simulink model "ex1"  (R2020a)
settings: Solver=VariableStepAuto  StartTime=0.0  StopTime=10.0  RelTol=1e-3
undefined symbols (not defined in the file or in its folder): DiscIntNeverNeededParam, dz, nz
libraries: simulink x1

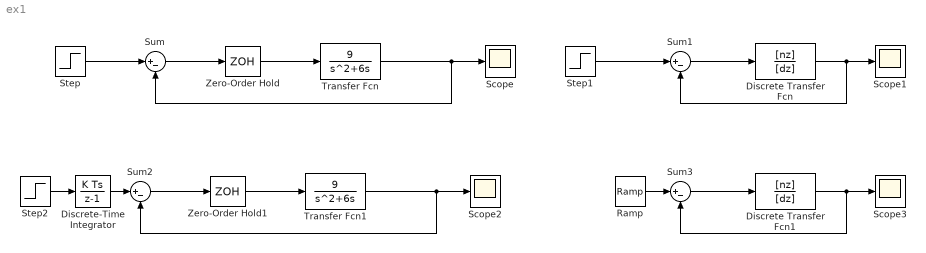
== system ex1 ==
  Discrete Transfer Fcn : DiscreteTransferFcn  Numerator=[nz]  Denominator=[dz]  SampleTime=0.1
  Discrete Transfer Fcn1 : DiscreteTransferFcn  Numerator=[nz]  Denominator=[dz]  SampleTime=0.1
  Discrete-Time Integrator : DiscreteIntegrator  SampleTime=-1  ICPrevOutput=DiscIntNeverNeededParam  ICPrevScaledInput=DiscIntNeverNeededParam
  Ramp : simulink/Sources/Ramp  slope=1  start=0  InitialOutput=0
  Scope{,1..3} (4 alike) : Scope
  Step : Step  SampleTime=0.1
  Step1 : Step  SampleTime=0.1
  Step2 : Step  SampleTime=0.1
  Sum{,1..3} (4 alike) : Sum  Inputs=|+-  SampleTime=0.1
  Transfer Fcn : TransferFcn  Numerator=[9]  Denominator=[1 6 0]
  Transfer Fcn1 : TransferFcn  Numerator=[9]  Denominator=[1 6 0]
  Zero-Order Hold : ZeroOrderHold  SampleTime=-1
  Zero-Order Hold1 : ZeroOrderHold  SampleTime=-1
  wires:
  Zero-Order Hold/1 -> Transfer Fcn/1
  Step/1 -> Sum/1
  Sum/1 -> Zero-Order Hold/1
  Transfer Fcn/1 -> Sum/2, Scope/1
  Step1/1 -> Sum1/1
  Sum1/1 -> Discrete Transfer Fcn/1
  Discrete Transfer Fcn/1 -> Sum1/2, Scope1/1
  Transfer Fcn1/1 -> Sum2/2, Scope2/1
  Zero-Order Hold1/1 -> Transfer Fcn1/1
  Sum2/1 -> Zero-Order Hold1/1
  Discrete Transfer Fcn1/1 -> Sum3/2, Scope3/1
  Sum3/1 -> Discrete Transfer Fcn1/1
  Ramp/1 -> Sum3/1
  Step2/1 -> Discrete-Time Integrator/1
  Discrete-Time Integrator/1 -> Sum2/1
